simulink model "FBBSC_7dof"  (R2024a)
settings: Solver=ode4  StartTime=0.0  StopTime=20  FixedStep=0.01  RelTol=1e-3
model workspace (MAT data in the model file):
  e2 = Simulink.Signal
  e2.DataType = 'auto'
  e2.Dimensions = [4 1]
  e2.DimensionsMode = 'Fixed'
  e2.Complexity = 'auto'
  e2.SampleTime = -1
  e2.SamplingMode = 'auto'
libraries: aerolibconvert2 x20
settings Model: Creator=hp  LastModifiedBy=somesh
settings SolverCC: ZeroCrossAlgorithm=Adaptive
settings DataIOCC: ReturnWorkspaceOutputs=off
settings DebuggingCC: IgnoredZcDiagnostic=none  UnderSpecifiedDimensionMsg=warning
settings RTWCC: GPUComputeCapability=3.5

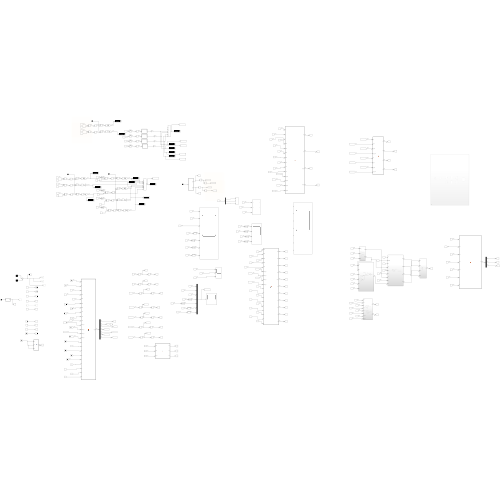
[thumbnail: Simulink's stored preview of the top-level diagram]
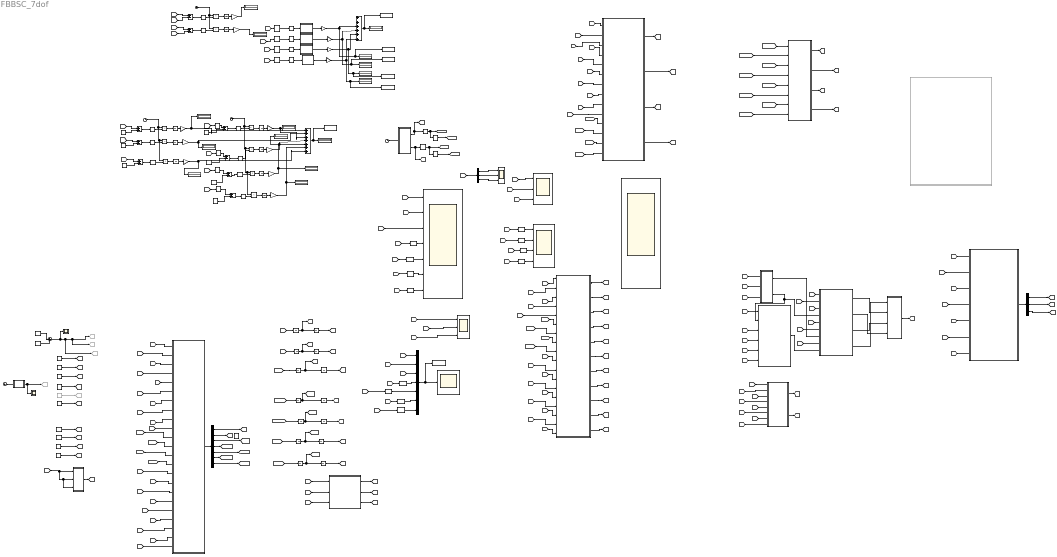
== system FBBSC_7dof ==
  Abs{,1..12} (13 alike) : Abs  SaturateOnIntegerOverflow=off
  Angle Conversion{,1..19} (20 alike) : aerolibconvert2/Angle Conversion  IU=rad  OU=deg
  Clock{,1,5,7..8} (5 alike) : Clock
  Constant : Constant  Value=6.1
  Constant1 : Constant  Value=15.6
  Constant11 : Constant  Value=0.5
  Constant12 : Constant  Value=0.6
  Constant{6..8,13,48..49} (6 alike) : Constant  Value=0
  Constant15 : Constant  Value=0.38
  Constant16 : Constant  Value=6.5
  Constant17 : Constant  Value=0.62
  Constant2 : Constant  Value=2
  Constant3 : Constant
  Constant4 : Constant  Commented=on  Value=0.5
  Constant5 : Constant  Value=0.5
  Constant9 : Constant  Value=0.7
  Demux : Demux  Outputs=7
  Demux1 : Demux  Outputs=3
  Demux3 : Demux  Outputs=3
  Derivative{,1..3} (4 alike) : Derivative
  Display{1..4,25,28..29,39,53..59} (15 alike) : Display
  Gain{,1..12} (13 alike) : Gain
  Goto18 : Goto  Commented=on  GotoTag=Fx
  Goto19 : Goto  Commented=on  GotoTag=Fy
  Goto24 : Goto  Commented=on  GotoTag=l1
  Goto52 : Goto  Commented=on  GotoTag=Fz
  Goto61 : Goto  Commented=on  GotoTag=m2
  Integrator{,1..7,12..20,22} (18 alike) : Integrator
  Integrator{8..11} (4 alike) : Integrator  WrapState=on  WrappedStateUpperValue=pi/2  WrappedStateLowerValue=-pi/2
  Integrator21 : Integrator  InitialCondition=0.5
  MATLAB Function : MATLAB Function  TreatAsAtomicUnit=on
  MATLAB Function1 : MATLAB Function  TreatAsAtomicUnit=on
  MATLAB Function13 : MATLAB Function  TreatAsAtomicUnit=on
  MATLAB Function14 : MATLAB Function  TreatAsAtomicUnit=on
  MATLAB Function16 : MATLAB Function  TreatAsAtomicUnit=on
  MATLAB Function17 : MATLAB Function  TreatAsAtomicUnit=on
  MATLAB Function2 : MATLAB Function  TreatAsAtomicUnit=on
  MATLAB Function20 : MATLAB Function  TreatAsAtomicUnit=on
  MATLAB Function3 : MATLAB Function  TreatAsAtomicUnit=on
  MATLAB Function4 : MATLAB Function  TreatAsAtomicUnit=on
  MATLAB Function5 : MATLAB Function  TreatAsAtomicUnit=on
  MATLAB Function6 : MATLAB Function  TreatAsAtomicUnit=on
  MATLAB Function7 : MATLAB Function  TreatAsAtomicUnit=on
  Mux12 : Mux  Inputs=7
  Product{,1..8} (9 alike) : Product
  Pulse Generator : DiscretePulseGenerator  PulseType=Time based  Amplitude=20  Period=100  PhaseDelay=1
  Pulse Generator1 : DiscretePulseGenerator  PulseType=Time based  Amplitude=-20  Period=100  PhaseDelay=2
  Scope : Scope  NumInputPorts=7
  Scope1 : Scope
  Scope13 : Scope
  Scope2 : Scope
  Scope3 : Scope  NumInputPorts=3
  Scope4 : Scope  NumInputPorts=3
  Scope5 : Scope  NumInputPorts=7
  Scope6 : Scope  NumInputPorts=4
  Scope9 : Scope  NumInputPorts=3
  Subsystem : Subsystem
  Subsystem1 : Subsystem
  Subsystem2 : Subsystem
  Subsystem3 : Subsystem
  Subsystem4 : Subsystem
  Subsystem5 : Subsystem  Commented=on
  Subtract{1..5,16..17,19..20} (9 alike) : Sum  Inputs=+-
  Sum : Sum  Inputs=|+++++++
  Sum2 : Sum  Inputs=|++
  Sum4 : Sum  Inputs=|++++++
  To Workspace : ToWorkspace  VariableName=theta_m  SampleTime=-1
  To Workspace1 : ToWorkspace  VariableName=ITAE  SampleTime=-1
  To Workspace2 : ToWorkspace  VariableName=theta_m1  SampleTime=-1
  To Workspace20 : ToWorkspace  VariableName=values  SaveFormat=Timeseries  SampleTime=-1
  To Workspace3 : ToWorkspace  VariableName=theta_m2  SampleTime=-1
  To Workspace4 : ToWorkspace  VariableName=theta_m3  SampleTime=-1
  To Workspace5 : ToWorkspace  VariableName=theta_m4  SampleTime=-1
  wires:
  [x_ddot] -> Integrator/1
  Integrator/1 -> Integrator6/1, [x_dot]
  [y_ddot] -> Integrator1/1
  Integrator1/1 -> Integrator7/1, [y_dot]
  [theta1_ddot] -> Integrator2/1
  Integrator2/1 -> Integrator8/1, [theta1_dot]
  [theta2_ddot] -> Integrator3/1
  Integrator3/1 -> Integrator9/1, [theta2_dot]
  [theta3_ddot] -> Integrator4/1
  Integrator4/1 -> Integrator10/1, [theta3_dot]
  [theta4_ddot] -> Integrator5/1
  Integrator5/1 -> Integrator11/1, [theta4_dot]
  Integrator6/1 -> [x]
  Integrator7/1 -> [y]
  Integrator8/1 -> [theta1]
  Integrator9/1 -> [theta2]
  Integrator10/1 -> [theta3]
  Integrator11/1 -> [theta4]
  [theta1] -> MATLAB Function/4(theta1)
  [theta2] -> MATLAB Function/5(theta2)
  [theta3] -> MATLAB Function/6(theta3)
  [theta4] -> MATLAB Function/7(theta4)
  [theta1_dot] -> MATLAB Function/11(theta1_dot)
  [theta2_dot] -> MATLAB Function/12(theta2_dot)
  [theta3_dot] -> MATLAB Function/13(theta3_dot)
  [theta4_dot] -> MATLAB Function/14(theta4_dot)
  Pulse Generator1/1 -> Sum2/2
  Pulse Generator/1 -> Sum2/1
  Sum2/1 -> Scope1/1, Goto52/1, Goto19/1, Goto18/1
  [m1] -> MATLAB Function/15(m1)
  [m2] -> MATLAB Function/16(m2)
  [M1] -> MATLAB Function/17(M1)
  [M2] -> MATLAB Function/18(M2)
  [l1] -> MATLAB Function/19(l1)
  [l2] -> MATLAB Function/20(l2)
  Constant/1 -> [M1]
  Constant1/1 -> [M2]
  Constant2/1 -> [m1]
  Constant3/1 -> [m2]
  Constant4/1 -> Goto24/1
  Constant5/1 -> [l2]
  Subtract16/1 -> Abs/1
  Integrator13/1 -> Gain3/1
  Constant7/1 -> Subtract20/2
  Gain2/1 -> Sum/3, Display39/1
  Integrator15/1 -> Gain5/1
  Gain1/1 -> Display25/1, Sum/2
  Product1/1 -> Integrator17/1
  Abs/1 -> Product/2
  [y] -> Subtract17/1
  Product2/1 -> Integrator14/1
  Subtract20/1 -> Abs4/1
  Abs2/1 -> Product2/2
  Abs3/1 -> Product3/2
  Gain5/1 -> Sum/6, Display29/1
  Abs5/1 -> Product5/2
  Integrator17/1 -> Gain1/1
  Clock8/1 -> Product5/1, Product2/1, Product4/1, Product3/1
  Gain3/1 -> Display1/1, Sum/4
  Subtract1/1 -> Abs2/1
  Constant48/1 -> Subtract1/2
  Integrator16/1 -> Gain/1
  Gain/1 -> Sum/1, Display3/1
  Product4/1 -> Integrator13/1
  Integrator14/1 -> Gain4/1
  Constant6/1 -> Subtract19/2
  Integrator12/1 -> Gain2/1
  Constant12/1 -> Subtract17/2
  Product5/1 -> Integrator15/1
  Subtract2/1 -> Abs5/1
  Abs4/1 -> Product4/2
  Product/1 -> Integrator16/1
  Gain4/1 -> Display28/1, Sum/5
  [x] -> Subtract16/1
  Constant49/1 -> Subtract2/2
  Subtract17/1 -> Abs1/1
  Constant11/1 -> Subtract16/2
  Sum/1 -> Display4/1, To Workspace1/1
  Product3/1 -> Integrator12/1
  Abs1/1 -> Product1/2
  [theta2] -> Angle Conversion9/1
  Gain11/1 -> Sum4/6, To Workspace5/1, Display56/1
  Subtract4/1 -> Abs7/1
  Gain10/1 -> To Workspace4/1, Display58/1, Sum4/5
  Subtract3/1 -> Abs6/1
  Abs11/1 -> MATLAB Function2/1(u)
  MATLAB Function20/1(y) -> Gain11/1
  [x_d] -> Subtract3/2
  [y_d] -> Subtract4/2
  [x] -> Subtract3/1
  MATLAB Function2/1(y) -> Gain8/1
  [theta4] -> Angle Conversion11/1
  Clock5/1 -> Product7/1, Product6/1
  MATLAB Function16/1(y) -> Gain10/1
  [theta3] -> Angle Conversion10/1
  Abs6/1 -> Product6/2
  [y] -> Subtract4/1
  Abs9/1 -> MATLAB Function16/1(u)
  Integrator18/1 -> Gain6/1
  Sum4/1 -> To Workspace/1, Display59/1
  Abs10/1 -> MATLAB Function20/1(u)
  MATLAB Function13/1(y) -> Gain9/1
  Product7/1 -> Integrator19/1
  Abs8/1 -> MATLAB Function13/1(u)
  [theta1] -> Angle Conversion8/1
  Gain7/1 -> Display54/1
  Product6/1 -> Integrator18/1
  Gain6/1 -> Display57/1
  Abs7/1 -> Product7/2
  Gain9/1 -> Sum4/4, To Workspace3/1, Display55/1
  Integrator19/1 -> Gain7/1
  Subtract19/1 -> Abs3/1
  [theta1] -> Angle Conversion4/1
  Angle Conversion4/1 -> Subtract19/1
  [theta2] -> Angle Conversion5/1
  Angle Conversion5/1 -> Subtract20/1
  [theta3] -> Angle Conversion6/1
  Angle Conversion6/1 -> Subtract1/1
  [theta4] -> Angle Conversion7/1
  Angle Conversion7/1 -> Subtract2/1
  Angle Conversion8/1 -> Abs11/1
  Angle Conversion9/1 -> Abs8/1
  Angle Conversion10/1 -> Abs9/1
  Angle Conversion11/1 -> Abs10/1
  [theta3] -> Angle Conversion16/1
  [theta1] -> Angle Conversion14/1
  Mux12/1 -> Scope2/1, To Workspace20/1
  [theta2] -> Angle Conversion15/1
  [theta4] -> Angle Conversion17/1
  [x] -> Scope/1
  [y] -> Scope/2
  [theta4] -> Angle Conversion3/1
  [theta3] -> Angle Conversion2/1
  [theta1] -> Angle Conversion/1
  [theta2] -> Angle Conversion1/1
  [x] -> MATLAB Function3/1(x)
  [y] -> MATLAB Function3/2(y)
  [theta1] -> MATLAB Function3/4(theta1)
  [theta2] -> MATLAB Function3/5(theta2)
  [theta3] -> MATLAB Function3/6(theta3)
  [theta4] -> MATLAB Function3/7(theta4)
  [x_dot] -> MATLAB Function3/8(x_dot)
  [y_dot] -> MATLAB Function3/9(y_dot)
  [theta1_dot] -> MATLAB Function3/11(theta1_dot)
  [theta2_dot] -> MATLAB Function3/12(theta2_dot)
  [theta3_dot] -> MATLAB Function3/13(theta3_dot)
  [theta4_dot] -> MATLAB Function3/14(theta4_dot)
  MATLAB Function3/1(qx) -> [qx]
  MATLAB Function3/2(qs) -> [qs]
  MATLAB Function3/3(qx_dot) -> [qx_dot]
  MATLAB Function3/4(qs_dot) -> [qs_dot]
  [qx_dot] -> MATLAB Function5/7(qx_dot)
  MATLAB Function5/3(e3) -> [e3]
  [qs_dot] -> MATLAB Function5/3(qs_dot)
  [qs_d] -> MATLAB Function5/2(qs_d)
  [qx] -> MATLAB Function5/5(qx)
  MATLAB Function5/4(e4) -> [e4]
  MATLAB Function5/2(e2) -> [e2]
  [qx_d] -> MATLAB Function5/6(qx_d)
  MATLAB Function5/1(e1) -> [e1]
  [qs_d_Dot] -> MATLAB Function5/4(qs_d_dot)
  [qs] -> MATLAB Function5/1(qs)
  [qx_d_Dot] -> MATLAB Function5/8(qx_d_dot)
  [Fx] -> MATLAB Function/1(Fx)
  [Fy] -> MATLAB Function/2(Fy)
  MATLAB Function/1(q_ddot) -> Demux/1
  [x_dot] -> MATLAB Function/8(x_dot)
  [y_dot] -> MATLAB Function/9(y_dot)
  [e3] -> Subsystem1/5(e3)
  MATLAB Function14/4(mss) -> [mss]
  MATLAB Function14/5(mss_I) -> [mss_I]
  MATLAB Function14/3(msx) -> [msx]
  MATLAB Function14/6(cxx) -> [cxx]
  [theta1_dot] -> MATLAB Function14/6(theta1_dot)
  [theta2_dot] -> MATLAB Function14/7(theta2_dot)
  [m1] -> MATLAB Function14/10(m1)
  [m2] -> MATLAB Function14/11(m2)
  [theta4] -> MATLAB Function14/4(theta4)
  [theta1] -> MATLAB Function14/1(theta1)
  [l2] -> MATLAB Function14/15(l2)
  MATLAB Function14/11(G2) -> [G2]
  MATLAB Function14/2(mxs) -> [mxs]
  [K] -> Subsystem/8(K)
  [M2] -> MATLAB Function14/13(M2)
  MATLAB Function14/8(csx) -> [csx]
  [K] -> Subsystem1/4(K)
  Subsystem/2(T4) -> Subsystem2/4(T4)
  MATLAB Function14/10(G1) -> [G1]
  [theta4_dot] -> MATLAB Function14/9(theta4_dot)
  [e2] -> Subsystem/6(e2)
  MATLAB Function14/7(cxs) -> [cxs]
  [qs_dot] -> Subsystem3/8(qs_dot)
  Subsystem4/1(ff) -> Subsystem/7(ff)
  Subsystem3/1(hx) -> [hx]
  Subsystem/3(T3) -> Subsystem2/3(T3)
  [theta3] -> MATLAB Function14/3(theta3)
  [css] -> Subsystem3/5(css)
  Subsystem/1(T2) -> Subsystem2/2(T2)
  [e4] -> Subsystem1/3(e4)
  [lambda] -> Subsystem/2(lambda)
  MATLAB Function14/9(css) -> [css]
  [G2] -> Subsystem3/6(G2)
  Subsystem/4(T1) -> Subsystem2/1(T1)
  [G1] -> Subsystem3/3(G1)
  Subsystem3/2(hs) -> [hs]
  MATLAB Function14/1(mxx) -> [mxx]
  [csx] -> Subsystem3/4(csx)
  [c2] -> Subsystem/3(c2)
  [l1] -> MATLAB Function14/14(l1)
  [qx_dot] -> Subsystem3/7(qx_dot)
  [e1] -> Subsystem1/6(e1)
  Subsystem2/1(U) -> [U]
  [cxx] -> Subsystem3/1(cxx)
  [hs] -> Subsystem4/2(hs)
  Subsystem1/1(z1) -> Subsystem/9(z1)
  [msx] -> Subsystem4/3(msx)
  [e4] -> Subsystem/5(e4)
  [mss_I] -> Subsystem4/1(mss_I)
  [M1] -> MATLAB Function14/12(M1)
  [e2] -> Subsystem1/1(e2)
  [mxx] -> MATLAB Function17/2(mxx)
  [U] -> MATLAB Function17/1(U)
  [msx] -> MATLAB Function17/5(msx)
  [c1] -> Subsystem/1(c1)
  MATLAB Function17/1(tau) -> Demux1/1
  [hs] -> MATLAB Function17/7(hs)
  [mss] -> MATLAB Function17/4(mss)
  Subsystem4/2(gf) -> Subsystem/4(gf), Subsystem1/2(gf)
  [theta2] -> MATLAB Function14/2(theta2)
  [theta3_dot] -> MATLAB Function14/8(theta3_dot)
  [mxs] -> MATLAB Function17/3(mxs)
  [cxs] -> Subsystem3/2(cxs)
  [hx] -> MATLAB Function17/6(hx)
  Gain8/1 -> To Workspace2/1, Display53/1, Sum4/3
  [Fx] -> Scope3/1
  [Fy] -> Scope3/2
  MATLAB Function1/1(K) -> [K]
  MATLAB Function4/1(m2) -> Goto61/1, Scope13/1
  Clock1/1 -> MATLAB Function4/1(t)
  [k] -> MATLAB Function1/3(k3), MATLAB Function1/2(k2), MATLAB Function1/1(k1)
  [x_dot] -> MATLAB Function7/1(x_dot)
  [y_dot] -> MATLAB Function7/2(y_dot)
  MATLAB Function7/1(Frx) -> [Frx]
  MATLAB Function7/2(Fry) -> [Fry]
  [Frx] -> MATLAB Function/21(Frx)
  [Fry] -> MATLAB Function/22(Fry)
  [Frx] -> MATLAB Function14/16(Frx)
  [Fry] -> MATLAB Function14/17(Fry)
  Constant15/1 -> [c1]
  Constant16/1 -> [c2]
  Constant17/1 -> [k]
  Constant13/1 -> [lambda]
  [Frz] -> MATLAB Function14/18(Frz)
  [Fz] -> MATLAB Function/3(Fz)
  [l1_dot] -> MATLAB Function7/3(l1_dot)
  MATLAB Function7/3(Frz) -> [Frz]
  Demux/7 -> [theta4_ddot]
  Demux/6 -> [theta3_ddot]
  Demux/5 -> [theta2_ddot]
  Demux/4 -> [theta1_ddot]
  Demux/2 -> [y_ddot]
  Demux/1 -> [x_ddot]
  [l1_dot] -> MATLAB Function/10(l1_dot)
  [Frz] -> MATLAB Function/23(Frz)
  [l1_ddot] -> Integrator20/1
  Integrator20/1 -> [l1_dot], Integrator21/1
  Integrator21/1 -> [l1]
  [Fz] -> Scope3/3
  [x] -> Mux12/1
  [y] -> Mux12/2
  [l1] -> Mux12/3
  Angle Conversion14/1 -> Mux12/4
  Angle Conversion15/1 -> Mux12/5
  Angle Conversion16/1 -> Mux12/6
  Angle Conversion17/1 -> Mux12/7
  [l1_dot] -> MATLAB Function14/5(l1_dot)
  [l1] -> Scope/3
  Angle Conversion/1 -> Scope/4
  Angle Conversion1/1 -> Scope/5
  Angle Conversion2/1 -> Scope/6
  Angle Conversion3/1 -> Scope/7
  [l1] -> MATLAB Function3/3(l)
  [l1_dot] -> MATLAB Function3/10(l_dot)
  Demux1/1 -> [Fx]
  Demux1/2 -> [Fy]
  Demux1/3 -> [Fz]
  Demux/3 -> [l1_ddot]
  Abs12/1 -> Product8/2
  Subtract5/1 -> Abs12/1
  Constant9/1 -> Subtract5/2
  Clock7/1 -> Product8/1, Product1/1, Product/1
  Integrator22/1 -> Gain12/1
  [l1] -> Subtract5/1
  Product8/1 -> Integrator22/1
  Gain12/1 -> Sum/7, Display2/1
  [theta1] -> Angle Conversion12/1
  [theta2] -> Angle Conversion13/1
  [theta3] -> Angle Conversion18/1
  [theta4] -> Angle Conversion19/1
  [x] -> Scope4/1
  [y] -> Scope4/2
  [l1] -> Scope4/3
  Angle Conversion12/1 -> Scope6/1
  Angle Conversion13/1 -> Scope6/2
  Angle Conversion18/1 -> Scope6/3
  Angle Conversion19/1 -> Scope6/4
  Demux3/3 -> Scope9/3
  [qx_d] -> Demux3/1
  Derivative1/1 -> [qs_d_DDot]
  Derivative2/1 -> Derivative3/1, [qx_d_Dot]
  MATLAB Function6/1(qs_d) -> Derivative/1, [qs_d]
  Demux3/1 -> Scope9/1
  Demux3/2 -> Scope9/2
  Clock/1 -> MATLAB Function6/1(t)
  Derivative/1 -> Derivative1/1, [qs_d_Dot]
  Derivative3/1 -> [qx_d_DDot]
  MATLAB Function6/2(qx_d) -> [qx_d], Derivative2/1

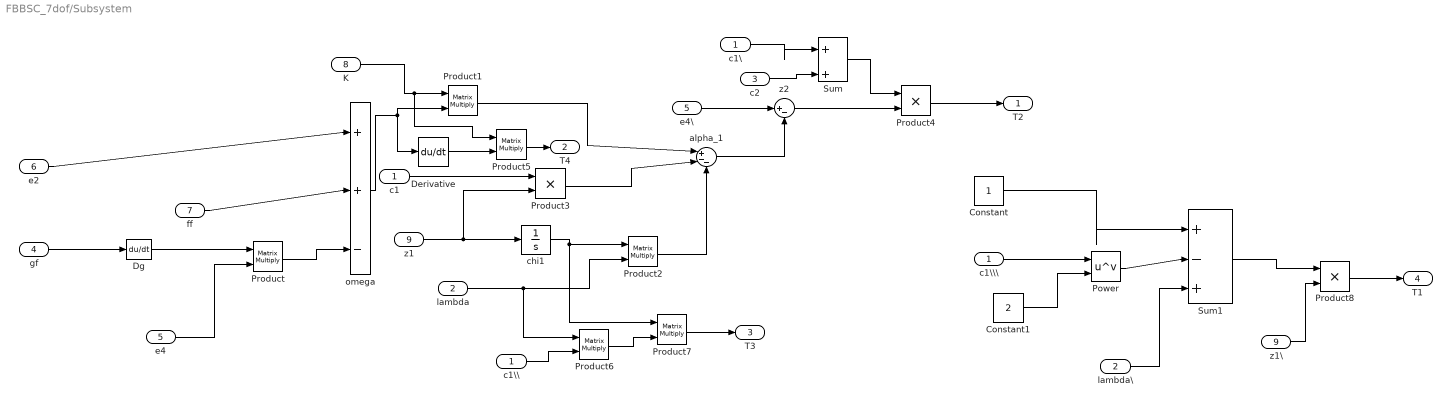
== system FBBSC_7dof/Subsystem ==
  c1 : Inport
  lambda : Inport  Port=2
  c2 : Inport  Port=3
  gf : Inport  Port=4  PortDimensions=[4 3]
  e4 : Inport  Port=5  PortDimensions=[3 1]
  e2 : Inport  Port=6  PortDimensions=[4 1]
  ff : Inport  Port=7  PortDimensions=[4 1]
  K : Inport  Port=8  PortDimensions=[3 4]
  z1 : Inport  Port=9  PortDimensions=[3 1]
  Constant : Constant
  Constant1 : Constant  Value=2
  Derivative : Derivative
  Dg : Derivative
  Power : Math  Operator=pow
  Product{,1..2,5..7} (6 alike) : Product  Multiplication=Matrix(*)
  Product3 : Product
  Product4 : Product
  Product8 : Product
  Sum : Sum  Inputs=|++
  Sum1 : Sum  Inputs=|+-+
  alpha_1 : Sum  Inputs=|+--
  c1\ : InportShadow
  c1\\ : InportShadow
  c1\\\ : InportShadow
  chi1 : Integrator
  e4\ : InportShadow  Port=5  PortDimensions=[3 1]
  lambda\ : InportShadow  Port=2
  omega : Sum  Inputs=|++-
  z1\ : InportShadow  Port=9  PortDimensions=[3 1]
  z2 : Sum  Inputs=|+-
  T2 : Outport  PortDimensions=[3 1]
  T4 : Outport  Port=2  PortDimensions=[3 1]
  T3 : Outport  Port=3  PortDimensions=[3 1]
  T1 : Outport  Port=4  PortDimensions=[3 1]
  wires:
  Dg/1 -> Product/1
  Product/1 -> omega/3
  omega/1 -> Product1/2, Derivative/1
  chi1/1 -> Product7/1, Product2/1
  lambda/1 -> Product6/1, Product2/2
  c1/1 -> Product3/1
  Product1/1 -> alpha_1/1
  Product3/1 -> alpha_1/2
  Product2/1 -> alpha_1/3
  alpha_1/1 -> z2/2
  c1\/1 -> Sum/1
  c2/1 -> Sum/2
  Sum/1 -> Product4/1
  z2/1 -> Product4/2
  Product4/1 -> T2/1
  Derivative/1 -> Product5/2
  Product5/1 -> T4/1
  c1\\/1 -> Product6/2
  Product6/1 -> Product7/2
  Product7/1 -> T3/1
  c1\\\/1 -> Power/1
  Constant1/1 -> Power/2
  Constant/1 -> Sum1/1
  Power/1 -> Sum1/2
  lambda\/1 -> Sum1/3
  Sum1/1 -> Product8/1
  Product8/1 -> T1/1
  gf/1 -> Dg/1
  e4/1 -> Product/2
  e2/1 -> omega/1
  ff/1 -> omega/2
  K/1 -> Product5/1, Product1/1
  z1/1 -> chi1/1, Product3/2
  e4\/1 -> z2/1
  z1\/1 -> Product8/2

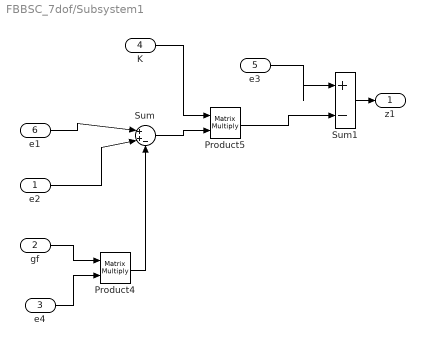
== system FBBSC_7dof/Subsystem1 ==
  e2 : Inport  PortDimensions=[4 1]
  gf : Inport  Port=2  PortDimensions=[4 3]
  e4 : Inport  Port=3  PortDimensions=[3 1]
  K : Inport  Port=4  PortDimensions=[3 4]
  e3 : Inport  Port=5  PortDimensions=[3 1]
  e1 : Inport  Port=6  PortDimensions=[4 1]
  Product4 : Product  Multiplication=Matrix(*)
  Product5 : Product  Multiplication=Matrix(*)
  Sum : Sum  Inputs=|++-
  Sum1 : Sum  Inputs=|+-
  z1 : Outport  PortDimensions=[3 1]
  wires:
  K/1 -> Product5/1
  gf/1 -> Product4/1
  e3/1 -> Sum1/1
  Product5/1 -> Sum1/2
  Sum/1 -> Product5/2
  e2/1 -> Sum/2
  e1/1 -> Sum/1
  e4/1 -> Product4/2
  Product4/1 -> Sum/3
  Sum1/1 -> z1/1

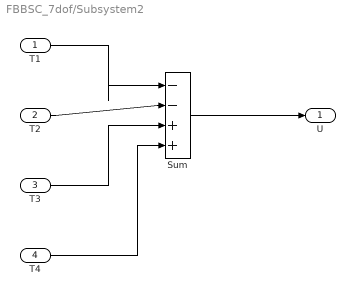
== system FBBSC_7dof/Subsystem2 ==
  T1 : Inport  PortDimensions=[3 1]
  T2 : Inport  Port=2  PortDimensions=[3 1]
  T3 : Inport  Port=3  PortDimensions=[3 1]
  T4 : Inport  Port=4  PortDimensions=[3 1]
  Sum : Sum  Inputs=|--++
  U : Outport  PortDimensions=[3 1]
  wires:
  T1/1 -> Sum/1
  T2/1 -> Sum/2
  T3/1 -> Sum/3
  T4/1 -> Sum/4
  Sum/1 -> U/1

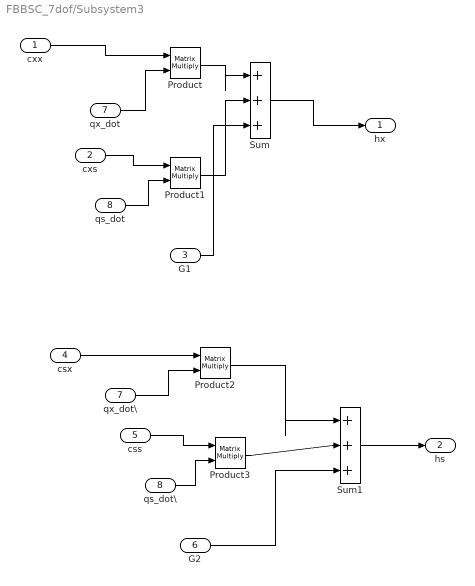
== system FBBSC_7dof/Subsystem3 ==
  cxx : Inport  PortDimensions=[3 3]
  cxs : Inport  Port=2  PortDimensions=[3 4]
  G1 : Inport  Port=3  PortDimensions=[3 1]
  csx : Inport  Port=4  PortDimensions=[4 3]
  css : Inport  Port=5  PortDimensions=[4 4]
  G2 : Inport  Port=6  PortDimensions=[4 1]
  qx_dot : Inport  Port=7  PortDimensions=[3 1]
  qs_dot : Inport  Port=8  PortDimensions=[4 1]
  Product{,1..3} (4 alike) : Product  Multiplication=Matrix(*)
  Sum : Sum  Inputs=|+++
  Sum1 : Sum  Inputs=|+++
  qs_dot\ : InportShadow  Port=8  PortDimensions=[4 1]
  qx_dot\ : InportShadow  Port=7  PortDimensions=[3 1]
  hx : Outport  PortDimensions=[3 1]
  hs : Outport  Port=2  PortDimensions=[4 1]
  wires:
  cxx/1 -> Product/1
  qx_dot/1 -> Product/2
  cxs/1 -> Product1/1
  qs_dot/1 -> Product1/2
  Product/1 -> Sum/1
  Product1/1 -> Sum/2
  G1/1 -> Sum/3
  Sum/1 -> hx/1
  Sum1/1 -> hs/1
  csx/1 -> Product2/1
  qx_dot\/1 -> Product2/2
  Product2/1 -> Sum1/1
  css/1 -> Product3/1
  qs_dot\/1 -> Product3/2
  Product3/1 -> Sum1/2
  G2/1 -> Sum1/3

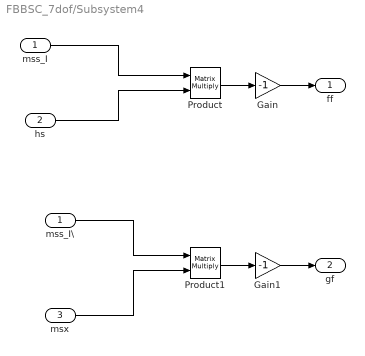
== system FBBSC_7dof/Subsystem4 ==
  mss_I : Inport  PortDimensions=[4 4]
  hs : Inport  Port=2  PortDimensions=[4 1]
  msx : Inport  Port=3  PortDimensions=[4 3]
  Gain : Gain  Gain=-1
  Gain1 : Gain  Gain=-1
  Product : Product  Multiplication=Matrix(*)
  Product1 : Product  Multiplication=Matrix(*)
  mss_I\ : InportShadow  PortDimensions=[4 4]
  ff : Outport  PortDimensions=[4 1]
  gf : Outport  Port=2  PortDimensions=[4 3]
  wires:
  hs/1 -> Product/2
  msx/1 -> Product1/2
  Product/1 -> Gain/1
  mss_I/1 -> Product/1
  mss_I\/1 -> Product1/1
  Product1/1 -> Gain1/1
  Gain/1 -> ff/1
  Gain1/1 -> gf/1

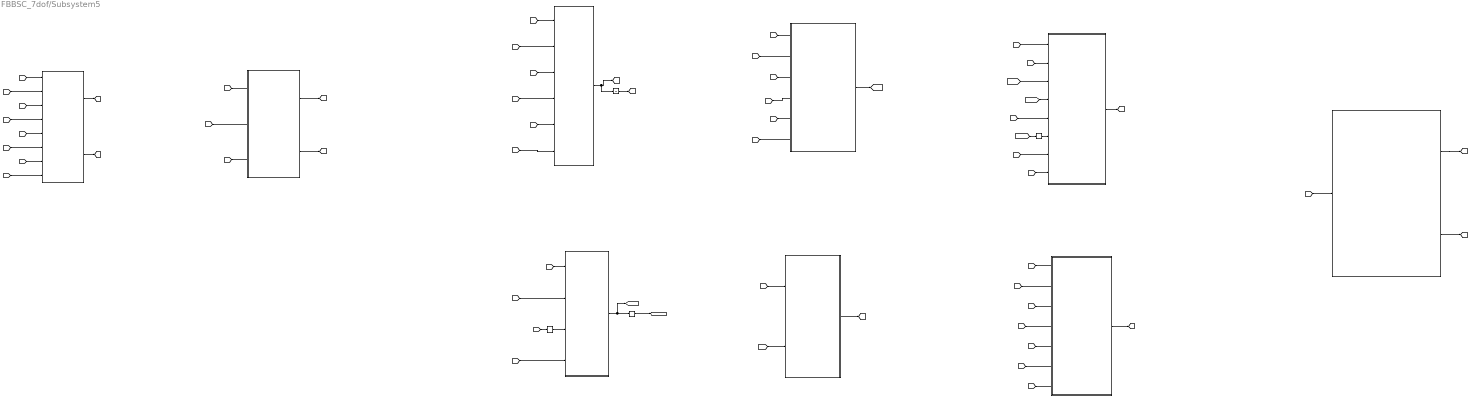
== system FBBSC_7dof/Subsystem5 ==
  Derivative4 : Derivative
  Integrator20 : Integrator
  MATLAB Function1 : MATLAB Function  TreatAsAtomicUnit=on
  MATLAB Function10 : MATLAB Function  TreatAsAtomicUnit=on
  MATLAB Function11 : MATLAB Function  TreatAsAtomicUnit=on
  MATLAB Function12 : MATLAB Function  TreatAsAtomicUnit=on
  MATLAB Function15 : MATLAB Function  TreatAsAtomicUnit=on
  MATLAB Function4 : MATLAB Function  TreatAsAtomicUnit=on
  MATLAB Function7 : MATLAB Function  TreatAsAtomicUnit=on
  MATLAB Function8 : MATLAB Function  TreatAsAtomicUnit=on
  MATLAB Function9 : MATLAB Function  TreatAsAtomicUnit=on
  Memory : Memory
  Memory3 : Memory
  wires:
  [c1] -> MATLAB Function11/1(c1)
  [z2] -> MATLAB Function11/4(z2)
  [lambda] -> MATLAB Function11/7(lambda)
  [msx] -> MATLAB Function12/5(msx)
  [chi1] -> MATLAB Function11/5(chi1)
  [Va] -> MATLAB Function15/1(tau)
  MATLAB Function8/1(Omega) -> Derivative4/1, [Omega]
  [c2] -> MATLAB Function11/2(c2)
  Memory/1 -> MATLAB Function11/6(omega_dot)
  [e2] -> MATLAB Function7/2(e2)
  [z1] -> MATLAB Function11/3(z1)
  [e4] -> MATLAB Function10/1(e4)
  MATLAB Function10/1(z2) -> [z2]
  [Dg] -> Memory3/1
  [Omega_dot] -> Memory/1
  [gf] -> MATLAB Function7/5(gf)
  [Omega] -> MATLAB Function9/6(Omega)
  Derivative4/1 -> [Omega_dot]
  [k] -> MATLAB Function7/6(k)
  MATLAB Function7/1(z1) -> Integrator20/1, [z1]
  [mxx] -> MATLAB Function12/2(mxx)
  [e4] -> MATLAB Function7/4(e4)
  [z1] -> MATLAB Function9/2(z1)
  [alpha_1] -> MATLAB Function10/2(alpha_1)
  MATLAB Function9/1(alpha_1) -> [alpha_1]
  MATLAB Function12/1(tau) -> [Va]
  MATLAB Function15/2(Fy) -> [Fy]
  [mxs] -> MATLAB Function12/3(mxs)
  [e1] -> MATLAB Function7/1(e1)
  Memory3/1 -> MATLAB Function8/3(Dg)
  MATLAB Function15/1(Fx) -> [Fx]
  [mss] -> MATLAB Function12/4(mss)
  MATLAB Function11/1(U) -> [U]
  Integrator20/1 -> [chi1]
  [ff] -> MATLAB Function8/2(ff)
  [k] -> MATLAB Function11/8(k)
  [e4] -> MATLAB Function8/4(e4)
  [e2] -> MATLAB Function8/1(e2)
  [hx] -> MATLAB Function12/6(hx)
  [e3] -> MATLAB Function7/3(e3)
  [chi1] -> MATLAB Function9/4(chi1)
  [k] -> MATLAB Function9/5(k)
  [lambda] -> MATLAB Function9/3(lambda)
  [hs] -> MATLAB Function12/7(hs)
  [U] -> MATLAB Function12/1(U)
  [c1] -> MATLAB Function9/1(c1)
  [G1] -> MATLAB Function1/3(G1)
  [qx_dot] -> MATLAB Function1/7(qx_dot)
  [msx] -> MATLAB Function4/2(msx)
  [csx] -> MATLAB Function1/4(csx)
  MATLAB Function4/1(ff) -> [ff]
  MATLAB Function4/2(gf) -> [gf]
  [qs_dot] -> MATLAB Function1/8(qs_dot)
  [mss] -> MATLAB Function4/1(mss)
  [css] -> MATLAB Function1/5(css)
  [cxs] -> MATLAB Function1/2(cxs)
  [hs] -> MATLAB Function4/3(hs)
  [G2] -> MATLAB Function1/6(G2)
  MATLAB Function1/2(hs) -> [hs]
  MATLAB Function1/1(hx) -> [hx]
  [cxx] -> MATLAB Function1/1(cxx)

== matlab function FBBSC_7dof/MATLAB Function13 ==
  settings: updateMethod=DISCRETE
  data: u input; y output
function y = fcn(u)
    persistent maxVal;
    
    % Check if maxVal is empty and initialize it if necessary
    if isempty(maxVal)
        maxVal = 0; % Initialize with negative infinity or another suitable value
    end
    
    % Update maxVal if the current input is greater
    if u > maxVal
        maxVal = u;
    end
    
    y = maxVal;
end

== matlab function FBBSC_7dof/MATLAB Function3 ==
  data: x input; qx output size=[3 1]; y input; l input; theta1 input; theta2 input; theta3 input; theta4 input; x_dot input; y_dot input; l_dot input; theta1_dot input; theta2_dot input; theta3_dot input; theta4_dot input; qs output size=[4 1]; qx_dot output size=[3 1]; qs_dot output size=[4 1]
function [qx, qs, qx_dot, qs_dot] = fcn(x, y, l, theta1, theta2, theta3, theta4,...
    x_dot, y_dot, l_dot, theta1_dot, theta2_dot, theta3_dot, theta4_dot)

qx = [x;y;l];
qs = [theta1;theta2;theta3;theta4];
qx_dot = [x_dot;y_dot; l_dot];
qs_dot = [theta1_dot;theta2_dot;theta3_dot;theta4_dot];

end

== matlab function FBBSC_7dof/Subsystem5/MATLAB Function4 ==
  data: mss input; ff output; msx input; hs input; gf output
function [ff, gf] = fcn(mss, msx, hs)

ff = -inv(mss)*hs;
gf = -inv(mss)*msx;

end

== matlab function FBBSC_7dof/MATLAB Function5 ==
  data: qs input size=[4 1]; e1 output size=[4 1]; qs_d input size=[4 1]; qs_dot input size=[4 1]; qs_d_dot input size=[4 1]; qx input size=[3 1]; qx_d input size=[3 1]; qx_dot input size=[3 1]; qx_d_dot input size=[3 1]; e2 output size=[4 1]; e3 output size=[3 1]; e4 output size=[3 1]
function [e1, e2, e3, e4] = fcn(qs, qs_d, qs_dot, qs_d_dot, qx, qx_d, qx_dot, qx_d_dot)


e1 = qs - qs_d;
e2 = qs_dot - qs_d_dot;
e3 = qx - qx_d;
e4 = qx_dot - qx_d_dot;

end

== matlab function FBBSC_7dof/MATLAB Function6 ==
  data: t input; qs_d output; qx_d output
function [qs_d, qx_d] = fcn(t)

qs_d = zeros(4,1);
qx_d = [0.5;0.6; 0.7];

% x0=0;
% y0=0;
% z0=0;
% x_d=0.5;
% y_d=0.6;
% z_d=0.7;
% kv= 0.4;
% ka = 0.4;
% epsilon = 1.5;
% k1 = (2*ka)/kv;
% k2 = (2*ka)/(kv^2);
% qx_d(1) = x0 + (x_d/2) + (kv/(2*k1))*(sqrt(1+(k1*t - epsilon)^2) - sqrt(1 + (k1*t - epsilon - k2*x_d)^2));
% qx_d(2) = y0 + (y_d/2) + (kv/(2*k1))*(sqrt(1+(k1*t - epsilon)^2) - sqrt(1 + (k1*t - epsilon - k2*y_d)^2));
% qx_d(3) = z0 + (z_d/2) + (kv/(2*k1))*(sqrt(1+(k1*t - epsilon)^2) - sqrt(1 + (k1*t - epsilon - k2*z_d)^2));

end


% if t >= 0 && t <= 20
%     
%   x_d = 0.02*t^2;
%   y_d = 0.03*t^2 ;
% 
%   
% elseif t >= 20 && t <= 60
%     
%   x_d = 8;
%   y_d = 12;
% 
%   
% elseif t >= 60 && t <= 80
%     
%   x_d = 8 + ((t - (60))^2)*0.03;
%   y_d = 12 + ((t-(60))^2)*0.02;
% 
%   
% else
%     x_d = 20;
%     y_d = 20;

== matlab function FBBSC_7dof/Subsystem5/MATLAB Function7 ==
  data: e1 input; z1 output; e2 input; e3 input; e4 input; gf input; k input
function z1  = fcn(e1, e2, e3, e4, gf, k)

K = [k, 0, 0, 0;
    0, k, 0, 0];

z1 = e3 - K*(e1 + e2 - gf*e4);




end

== matlab function FBBSC_7dof/Subsystem5/MATLAB Function8 ==
  data: e2 input; Omega output; ff input; Dg input; e4 input
function Omega = fcn(e2, ff, Dg, e4)

Omega = e2 + ff - Dg*e4;

end

== matlab function FBBSC_7dof/Subsystem5/MATLAB Function9 ==
  data: c1 input; alpha_1 output; z1 input; lambda input; chi1 input; k input; Omega input
function alpha_1 = fcn(c1, z1, lambda, chi1, k, Omega)


K = [k, 0, 0, 0;
    0, k, 0, 0];

alpha_1 = -c1.*z1 - lambda.*chi1 + K*Omega;

end

== matlab function FBBSC_7dof/Subsystem5/MATLAB Function10 ==
  data: e4 input; z2 output; alpha_1 input
function z2 = fcn(e4, alpha_1)

z2 = e4 - alpha_1;

end

== matlab function FBBSC_7dof/Subsystem5/MATLAB Function11 ==
  data: c1 input; c2 input; z1 input size=[2 1]; z2 input size=[2 1]; chi1 input size=[2 1]; omega_dot input size=[4 1]; lambda input; k input; U output size=[2 1]
function U  = fcn(c1, c2, z1, z2, chi1, omega_dot, lambda, k)

K = [k, 0, 0, 0;
    0, k, 0, 0];


U = - (1 - c1^2 + lambda).*z1 - (c1 + c2).*z2 + (lambda*c1).*chi1 + K*omega_dot;

end

== matlab function FBBSC_7dof/Subsystem5/MATLAB Function12 ==
  data: U input size=[2 1]; tau output; mxx input size=[2 2]; mxs input size=[2 4]; mss input size=[4 4]; msx input size=[4 2]; hx input size=[2 1]; hs input size=[4 1]
function tau  = fcn(U, mxx, mxs, mss, msx, hx, hs)

B = [1, 0; 0, 1];

tau = inv(B'*B)*B'*((mxx - mxs*inv(mss)*msx)*U + (hx - mxs*inv(mss)*hs));


end

== matlab function FBBSC_7dof/MATLAB Function14 ==
  data: theta1 input; theta2 input; theta3 input; theta4 input; l1_dot input; theta1_dot input; theta2_dot input; theta3_dot input; theta4_dot input; m1 input; m2 input; M1 input; M2 input; l1 input; l2 input; mxx output; mxs output; msx output; mss output; mss_I output; cxx output; cxs output; csx output; css output; G1 output; G2 output; Frx input; Fry input; Frz input
function [mxx, mxs, msx, mss, mss_I, cxx, cxs, csx, css, G1, G2]   = fcn(theta1, theta2, theta3, theta4,...
    l1_dot, theta1_dot, theta2_dot, theta3_dot, theta4_dot,...
    m1, m2, M1, M2, l1, l2, Frx, Fry, Frz)


g = 9.8;


% Mass matrix M(q)
M = zeros(7, 7);

% Define M matrix elements
M(1,1) = M1 + m1 + m2;
M(1,2) = 0;
M(1,3) = (m1 + m2) * sin(theta1) * cos(theta2);
M(1,4) = (m1 + m2) * l1 * cos(theta1) * cos(theta2);
M(1,5) = -(m1 + m2) * l1 * sin(theta1) * sin(theta2);
M(1,6) = m2 * l2 * cos(theta3) * cos(theta4);
M(1,7) = -m2 * l2 * sin(theta3) * sin(theta4);

M(2,1) = 0;
M(2,2) = M2 + m1 + m2;
M(2,3) = (m1 + m2) * sin(theta2);
M(2,4) = 0;
M(2,5) = (m1 + m2) * l1 * cos(theta2);
M(2,6) = 0;
M(2,7) = m2 * l2 * cos(theta4);

M(3,1) = (m1 + m2) * sin(theta1) * cos(theta2);
M(3,2) = (m1 + m2) * sin(theta2);
M(3,3) = m1 + m2;
M(3,4) = 0;
M(3,5) = 0;
M(3,6) = m2 * l2 * cos(theta2) * cos(theta4) * sin(theta1 - theta3);
M(3,7) = m2 * l2 * (sin(theta2) * cos(theta4) - cos(theta2) * sin(theta4) * cos(theta1 - theta3));

M(4,1) = (m1 + m2) * l1 * cos(theta1) * cos(theta2);
M(4,2) = 0;
M(4,3) = 0;
M(4,4) = (m1 + m2) * l1^2 * cos(theta2)^2;
M(4,5) = 0;
M(4,6) = m2*l1*l2*cos(theta2)*cos(theta4)*cos(theta1-theta3);
M(4,7) = m2*l1*l2*cos(theta2)*sin(theta4)*sin(theta1 - theta3);

M(5,1) = -(m1 + m2) * l1 * sin(theta1) * sin(theta2);
M(5,2) = (m1 + m2) * l1 * cos(theta2);
M(5,3) = 0;
M(5,4) = 0;
M(5,5) = (m1 + m2) * l1^2;
M(5,6) = -m2 * l1 * l2 * sin(theta2) * cos(theta4) * sin(theta1 - theta3);
M(5,7) = m2 * l1 * l2 * (cos(theta2) * cos(theta4) + sin(theta2) * sin(theta4) * cos(theta1 - theta3));

M(6,1) = m2 * l2 * cos(theta3) * cos(theta4);
M(6,2) = 0;
M(6,3) = m2 * l2 * cos(theta2) * cos(theta4) * sin(theta1 - theta3);
M(6,4) = m2*l1*l2*cos(theta2)*cos(theta4)*cos(theta1-theta3);
M(6,5) = -m2 * l1 * l2 * sin(theta2) * cos(theta4) * sin(theta1 - theta3);
M(6,6) = m2 * l2^2 * cos(theta4)^2;
M(6,7) = 0;

M(7,1) = -m2 * l2 * sin(theta3) * sin(theta4);
M(7,2) = m2 * l2 * cos(theta4);
M(7,3) = m2 * l2 * (sin(theta2) * cos(theta4) - cos(theta2) * sin(theta4) * cos(theta1 - theta3));
M(7,4) = m2*l1*l2*cos(theta2)*sin(theta4)*sin(theta1 - theta3);
M(7,5) = m2 * l1 * l2 * (cos(theta2) * cos(theta4) + sin(theta2) * sin(theta4) * cos(theta1 - theta3));
M(7,6) = 0;
M(7,7) = m2 * l2^2;

% spliting

mxx = M(1:3, 1:3);
mxs = M(1:3, 4:7);
msx = M(4:7, 1:3);
mss = M(4:7, 4:7);
mss_I = -inv(mss);

%%%%%%%%%%%%%%%%%%%%%%%%%%%%%%%%%%%%%%%%%%%%%%%%%%%%%%%%%%%%%%%%%%%%%%%%%%%%%%%%%%%%%%%%%%%%%%%%%%%%%%%%%%%%%%%%%%%%%%%%%%%%%%%%%%%%%%%%%%%%%%%%%%%%%%%%%%%%%%%%%%%%%%%%%%%%%%%%

% Coriolis matrix C(q, dq)
C = zeros(7, 7);

% Define C matrix elements
C(1,3) = (m1 + m2) * (cos(theta1) * cos(theta2) * theta1_dot - sin(theta1) * sin(theta2) * theta2_dot);
C(1,4) = (m1 + m2) * (cos(theta1) * cos(theta2) * l1_dot - l1 * sin(theta1) * sin(theta2) * theta1_dot - l1 * cos(theta1) * sin(theta2) * theta2_dot);
C(1,5) = -(m1 + m2) * (sin(theta1) * sin(theta2) * l1_dot + l1 * cos(theta1) * sin(theta2) * theta1_dot + l1 * sin(theta1) * cos(theta2) * theta2_dot);
C(1,6) = -m2 * l2 * (sin(theta3) * cos(theta4) * theta3_dot + cos(theta3) * sin(theta4) * theta4_dot);
C(1,7) = -m2 * l2 * (cos(theta3) * sin(theta4) * theta3_dot + sin(theta3) * cos(theta4) * theta4_dot);

C(2,3) = (m1 + m2) * cos(theta2) * theta2_dot;
C(2,5) = (m1 + m2) * (cos(theta2) * l1_dot - l1 * sin(theta2) * theta2_dot);
C(2,7) = -m2 * l2 * sin(theta4) * theta4_dot;

C(3,4) = -(m1 + m2) * l1 * cos(theta2)^2 * theta1_dot;
C(3,5) = -(m1 + m2) * l1 * theta2_dot;
C(3,6) = -m2 * l2 * (cos(theta2) * cos(theta4) * cos(theta1 - theta3) * theta3_dot + cos(theta2) * sin(theta4) * sin(theta1 - theta3) * theta4_dot);
C(3,7) = -m2 * l2 * (cos(theta2) * sin(theta4) * theta3_dot + sin(theta2) * sin(theta4) * theta4_dot + cos(theta2) * cos(theta4) * cos(theta1 - theta3) * theta4_dot);

C(4,3) = (m1 + m2) * l1 * cos(theta2)^2 * theta1_dot;
C(4,4) = (m1 + m2) * (l1 * cos(theta2)^2 * l1_dot - l1^2 * sin(theta2) * cos(theta2) * theta2_dot);
C(4,5) = -(m1 + m2) * l1^2 * sin(theta2) * cos(theta2) * theta1_dot;
C(4,6) = m2 * l1 * l2 * (cos(theta2) * cos(theta4) * sin(theta1 - theta3) * theta3_dot + cos(theta2) * sin(theta4) * cos(theta1 - theta3) * theta4_dot);
C(4,7) = m2 * l1 * l2 * (cos(theta2) * cos(theta4) * sin(theta1 - theta3) * theta4_dot + cos(theta2) * sin(theta4) * cos(theta1 - theta3) * theta3_dot);

C(5,3) = (m1 + m2) * l1 * theta2_dot;
C(5,4) = (m1 + m2) * l1^2 * sin(theta2) * cos(theta2) * theta1_dot;
C(5,5) = (m1 + m2) * l1 * l1_dot;
C(5,6) = m2 * l1 * l2 * (sin(theta2) * cos(theta4) * cos(theta1 - theta3) * theta3_dot + sin(theta2) * sin(theta4) * sin(theta1 - theta3) * theta4_dot);
C(5,7) = m2 * l1 * l2 * (sin(theta2) * sin(theta4) * sin(theta1 - theta3) * theta3_dot + sin(theta2) * cos(theta4) * cos(theta1 - theta3) * theta4_dot ...
    - cos(theta2) * sin(theta4) * theta4_dot);

C(6,3) = m2 * l2 * (cos(theta2) * cos(theta4) * cos(theta1 - theta3) * theta1_dot - sin(theta2) * cos(theta4) * sin(theta1 - theta3) * theta2_dot);
C(6,4) = m2 * l2 * (cos(theta2) * cos(theta4) * cos(theta1 - theta3) * l1_dot - l1 * cos(theta2) * cos(theta4) * sin(theta1 - theta3) ...
    * theta1_dot - l1 * sin(theta2) * cos(theta4) * cos(theta1 - theta3) * theta2_dot);
C(6,5) = -m2 * l2 * (sin(theta2) * cos(theta4) * sin(theta1 - theta3) * l1_dot + l1 * sin(theta2) * cos(theta4) * cos(theta1 - theta3) ...
    * theta1_dot + l1 * cos(theta2) * cos(theta4) * sin(theta1 - theta3) * theta2_dot);
C(6,6) = -m2 * l2^2 * sin(theta4) * cos(theta4) * theta4_dot;
C(6,7) = -m2 * l2^2 * sin(theta4) * cos(theta4) * theta3_dot;

C(7,3) = m2 * l2 * (cos(theta2) * sin(theta4) * sin(theta1 - theta3) * theta1_dot + sin(theta2) * sin(theta4) * cos(theta1 - theta3) * theta2_dot ...
    + cos(theta2) * cos(theta4) * theta2_dot);
C(7,4) = m2 * l2 * (cos(theta2) * sin(theta4) * sin(theta1 - theta3) * l1_dot + l1 * cos(theta2) * sin(theta4) * cos(theta1 - theta3) ...
    * theta1_dot - l1 * sin(theta2) * sin(theta4) * sin(theta1 - theta3)*theta2_dot);
C(7,5) = m2 * l2 * (cos(theta2)*cos(theta4)*l1_dot + sin(theta2)*sin(theta4)*cos(theta1 - theta3)*l1_dot - l1 * sin(theta2)*sin(theta4)...
    *sin(theta1 - theta3)*theta1_dot + l1*cos(theta2)*sin(theta4)*cos(theta1 - theta3)*theta2_dot - l1*sin(theta2)*cos(theta4)*theta2_dot);
C(7,6) = m2 * l2^2 * sin(theta4) * cos(theta4) * theta3_dot;

% spliting

cxx = C(1:3, 1:3);
cxs = C(1:3, 4:7);
csx = C(4:7, 1:3);
css = C(4:7, 4:7);

%%%%%%%%%%%%%%%%%%%%%%%%%%%%%%%%%%%%%%%%%%%%%%%%%%%%%%%%%%%%%%%%%%%%%%%%%%%%%%%%%%%%%%%%%%%%%%%%%%%%%%%%%%%%%%%%%%%%%%%%%%%%%%%%%%%%%%%%%%%%%%%%%%%%%%%%%%%%%%%%%%%%%%%%%%%%%%%%%%%%%

% Gravity with friction matrix
G = zeros(7, 1);

% Define G matrix elements
G(1,1) = Frx;
G(2,1) = Fry;
G(3,1) = Frz - (m1 + m2) * g * cos(theta1) * cos(theta2);
% G(3,1) = 0;
G(4,1) = (m1 + m2) * g * l1 * sin(theta1) * cos(theta2);
G(5,1) = (m1 + m2) * g * l1 * cos(theta1) * sin(theta2);
G(6,1) = m2 * g * l2 * sin(theta3) * cos(theta4);
G(7,1) = m2 * g * l2 * cos(theta3) * sin(theta4);

% spliting

G1 = G(1:3);
G2 = G(4:7);

%%%%%%%%%%%%%%%%%%%%%%%%%%%%%%%%%%%%%%%%%%%%%%%%%%%%%%%%%%%%%%%%%%%%%%%%%%%%%%%%%%%%%%%%%%%%%%%%%%%%%%%%%%%%%%%%%%%%%%%%%%%%%%%%%%%%%%%%%%%%%%%%%%%%%%%%%%%%%%%%%%%%%%%%%%%%%%%%%%%%%%


end

== matlab function FBBSC_7dof/Subsystem5/MATLAB Function15 ==
  data: tau input; Fx output; Fy output
function [Fx, Fy] = fcn(tau)

Fx = tau(1);
Fy = tau(2);
end

== matlab function FBBSC_7dof/MATLAB Function17 ==
  data: U input size=[3 1]; tau output size=[3 1]; mxx input size=[3 3]; mxs input size=[3 4]; mss input size=[4 4]; msx input size=[4 3]; hx input size=[3 1]; hs input size=[4 1]
function tau  = fcn(U, mxx, mxs, mss, msx, hx, hs)

B = [1, 0, 0;
    0, 1, 0;
    0, 0, 1];

tau = inv(B'*B)*B'*((mxx - mxs*inv(mss)*msx)*U + (hx - mxs*inv(mss)*hs));


end

== matlab function FBBSC_7dof/MATLAB Function1 ==
  data: k1 input; K output; k2 input; k3 input
function K = fcn(k1, k2, k3)

K = [k1, 0, 0, 0;
    0, k2, 0, 0;
    0, 0, k3, 0];

end

== matlab function FBBSC_7dof/MATLAB Function16 ==
  settings: updateMethod=DISCRETE
  data: u input; y output
function y = fcn(u)
    persistent maxVal;
    
    % Check if maxVal is empty and initialize it if necessary
    if isempty(maxVal)
        maxVal = 0; % Initialize with negative infinity or another suitable value
    end
    
    % Update maxVal if the current input is greater
    if u > maxVal
        maxVal = u;
    end
    
    y = maxVal;
end

== matlab function FBBSC_7dof/MATLAB Function4 ==
  data: t input; m2 output
function m2 = fcn(t)

if t>=0 && t<3
    m2 = 0.6;
else
    m2 = 0.2;

% m2 = 0.6;


end

== matlab function FBBSC_7dof/MATLAB Function7 ==
  data: x_dot input; Frx output; y_dot input; Fry output; l1_dot input; Frz output
function [Frx, Fry, Frz] = fcn(x_dot, y_dot, l1_dot)

frox = 0.6;
froy = 0.6;
epsilon_x = 0.6;
epsilon_y = 0.6;
krx = 0.1;
kry = 0.1;
dz = 0.1;

Frx = frox*tanh(x_dot/epsilon_x) - krx*abs(x_dot)*x_dot;
Fry = froy*tanh(y_dot/epsilon_y) - kry*abs(y_dot)*y_dot;
Frz = dz * l1_dot;
end

== matlab function FBBSC_7dof/MATLAB Function2 ==
  settings: updateMethod=DISCRETE
  data: u input; y output
function y = fcn(u)
    persistent maxVal;
    
    % Check if maxVal is empty and initialize it if necessary
    if isempty(maxVal)
        maxVal = 0; % Initialize with negative infinity or another suitable value
    end
    
    % Update maxVal if the current input is greater
    if u > maxVal
        maxVal = u;
    end
    
    y = maxVal;
end

== matlab function FBBSC_7dof/MATLAB Function20 ==
  settings: updateMethod=DISCRETE
  data: u input; y output
function y = fcn(u)
    persistent maxVal;
    
    % Check if maxVal is empty and initialize it if necessary
    if isempty(maxVal)
        maxVal = 0; % Initialize with negative infinity or another suitable value
    end
    
    % Update maxVal if the current input is greater
    if u > maxVal
        maxVal = u;
    end
    
    y = maxVal;
end

== matlab function FBBSC_7dof/Subsystem5/MATLAB Function1 ==
  data: cxx input size=[2 2]; hx output size=[2 1]; cxs input size=[2 4]; G1 input size=[2 1]; csx input size=[4 2]; css input size=[4 4]; G2 input size=[4 1]; qx_dot input size=[2 1]; qs_dot input size=[4 1]; hs output size=[4 1]
function [hx, hs] = fcn(cxx, cxs, G1, csx, css, G2, qx_dot, qs_dot)

hx = cxx*qx_dot + cxs*qs_dot + G1;
hs = csx*qx_dot + css*qs_dot + G2;

end

== matlab function FBBSC_7dof/MATLAB Function ==
  data: Fx input; Fy input; Fz input; theta1 input; theta2 input; theta3 input; theta4 input; x_dot input; y_dot input; l1_dot input; theta1_dot input; theta2_dot input; theta3_dot input; theta4_dot input; m1 input; m2 input; M1 input; M2 input; l1 input; l2 input; q_ddot output size=[7 1]; Frx input; Fry input; Frz input
function q_ddot   = fcn(Fx, Fy, Fz, theta1, theta2, theta3, theta4,...
    x_dot, y_dot, l1_dot, theta1_dot, theta2_dot, theta3_dot, theta4_dot,...
    m1, m2, M1, M2, l1, l2, Frx, Fry, Frz)

g = 9.8;


% Mass matrix M(q)
M = zeros(7, 7);

% Define M matrix elements
M(1,1) = M1 + m1 + m2;
M(1,2) = 0;
M(1,3) = (m1 + m2) * sin(theta1) * cos(theta2);
M(1,4) = (m1 + m2) * l1 * cos(theta1) * cos(theta2);
M(1,5) = -(m1 + m2) * l1 * sin(theta1) * sin(theta2);
M(1,6) = m2 * l2 * cos(theta3) * cos(theta4);
M(1,7) = -m2 * l2 * sin(theta3) * sin(theta4);

M(2,1) = 0;
M(2,2) = M2 + m1 + m2;
M(2,3) = (m1 + m2) * sin(theta2);
M(2,4) = 0;
M(2,5) = (m1 + m2) * l1 * cos(theta2);
M(2,6) = 0;
M(2,7) = m2 * l2 * cos(theta4);

M(3,1) = (m1 + m2) * sin(theta1) * cos(theta2);
M(3,2) = (m1 + m2) * sin(theta2);
M(3,3) = m1 + m2;
M(3,4) = 0;
M(3,5) = 0;
M(3,6) = m2 * l2 * cos(theta2) * cos(theta4) * sin(theta1 - theta3);
M(3,7) = m2 * l2 * (sin(theta2) * cos(theta4) - cos(theta2) * sin(theta4) * cos(theta1 - theta3));

M(4,1) = (m1 + m2) * l1 * cos(theta1) * cos(theta2);
M(4,2) = 0;
M(4,3) = 0;
M(4,4) = (m1 + m2) * l1^2 * cos(theta2)^2;
M(4,5) = 0;
M(4,6) = m2*l1*l2*cos(theta2)*cos(theta4)*cos(theta1-theta3);
M(4,7) = m2*l1*l2*cos(theta2)*sin(theta4)*sin(theta1 - theta3);

M(5,1) = -(m1 + m2) * l1 * sin(theta1) * sin(theta2);
M(5,2) = (m1 + m2) * l1 * cos(theta2);
M(5,3) = 0;
M(5,4) = 0;
M(5,5) = (m1 + m2) * l1^2;
M(5,6) = -m2 * l1 * l2 * sin(theta2) * cos(theta4) * sin(theta1 - theta3);
M(5,7) = m2 * l1 * l2 * (cos(theta2) * cos(theta4) + sin(theta2) * sin(theta4) * cos(theta1 - theta3));

M(6,1) = m2 * l2 * cos(theta3) * cos(theta4);
M(6,2) = 0;
M(6,3) = m2 * l2 * cos(theta2) * cos(theta4) * sin(theta1 - theta3);
M(6,4) = m2*l1*l2*cos(theta2)*cos(theta4)*cos(theta1-theta3);
M(6,5) = -m2 * l1 * l2 * sin(theta2) * cos(theta4) * sin(theta1 - theta3);
M(6,6) = m2 * l2^2 * cos(theta4)^2;
M(6,7) = 0;

M(7,1) = -m2 * l2 * sin(theta3) * sin(theta4);
M(7,2) = m2 * l2 * cos(theta4);
M(7,3) = m2 * l2 * (sin(theta2) * cos(theta4) - cos(theta2) * sin(theta4) * cos(theta1 - theta3));
M(7,4) = m2*l1*l2*cos(theta2)*sin(theta4)*sin(theta1 - theta3);
M(7,5) = m2 * l1 * l2 * (cos(theta2) * cos(theta4) + sin(theta2) * sin(theta4) * cos(theta1 - theta3));
M(7,6) = 0;
M(7,7) = m2 * l2^2;

% Coriolis matrix C(q, dq)
C = zeros(7, 7);

% Define C matrix elements
C(1,3) = (m1 + m2) * (cos(theta1) * cos(theta2) * theta1_dot - sin(theta1) * sin(theta2) * theta2_dot);
C(1,4) = (m1 + m2) * (cos(theta1) * cos(theta2) * l1_dot - l1 * sin(theta1) * sin(theta2) * theta1_dot - l1 * cos(theta1) * sin(theta2) * theta2_dot);
C(1,5) = -(m1 + m2) * (sin(theta1) * sin(theta2) * l1_dot + l1 * cos(theta1) * sin(theta2) * theta1_dot + l1 * sin(theta1) * cos(theta2) * theta2_dot);
C(1,6) = -m2 * l2 * (sin(theta3) * cos(theta4) * theta3_dot + cos(theta3) * sin(theta4) * theta4_dot);
C(1,7) = -m2 * l2 * (cos(theta3) * sin(theta4) * theta3_dot + sin(theta3) * cos(theta4) * theta4_dot);

C(2,3) = (m1 + m2) * cos(theta2) * theta2_dot;
C(2,5) = (m1 + m2) * (cos(theta2) * l1_dot - l1 * sin(theta2) * theta2_dot);
C(2,7) = -m2 * l2 * sin(theta4) * theta4_dot;

C(3,4) = -(m1 + m2) * l1 * cos(theta2)^2 * theta1_dot;
C(3,5) = -(m1 + m2) * l1 * theta2_dot;
C(3,6) = -m2 * l2 * (cos(theta2) * cos(theta4) * cos(theta1 - theta3) * theta3_dot + cos(theta2) * sin(theta4) * sin(theta1 - theta3) * theta4_dot);
C(3,7) = -m2 * l2 * (cos(theta2) * sin(theta4) * theta3_dot + sin(theta2) * sin(theta4) * theta4_dot + cos(theta2) * cos(theta4) * cos(theta1 - theta3) * theta4_dot);

C(4,3) = (m1 + m2) * l1 * cos(theta2)^2 * theta1_dot;
C(4,4) = (m1 + m2) * (l1 * cos(theta2)^2 * l1_dot - l1^2 * sin(theta2) * cos(theta2) * theta2_dot);
C(4,5) = -(m1 + m2) * l1^2 * sin(theta2) * cos(theta2) * theta1_dot;
C(4,6) = m2 * l1 * l2 * (cos(theta2) * cos(theta4) * sin(theta1 - theta3) * theta3_dot + cos(theta2) * sin(theta4) * cos(theta1 - theta3) * theta4_dot);
C(4,7) = m2 * l1 * l2 * (cos(theta2) * cos(theta4) * sin(theta1 - theta3) * theta4_dot + cos(theta2) * sin(theta4) * cos(theta1 - theta3) * theta3_dot);

C(5,3) = (m1 + m2) * l1 * theta2_dot;
C(5,4) = (m1 + m2) * l1^2 * sin(theta2) * cos(theta2) * theta1_dot;
C(5,5) = (m1 + m2) * l1 * l1_dot;
C(5,6) = m2 * l1 * l2 * (sin(theta2) * cos(theta4) * cos(theta1 - theta3) * theta3_dot + sin(theta2) * sin(theta4) * sin(theta1 - theta3) * theta4_dot);
C(5,7) = m2 * l1 * l2 * (sin(theta2) * sin(theta4) * sin(theta1 - theta3) * theta3_dot + sin(theta2) * cos(theta4) * cos(theta1 - theta3) * theta4_dot ...
    - cos(theta2) * sin(theta4) * theta4_dot);

C(6,3) = m2 * l2 * (cos(theta2) * cos(theta4) * cos(theta1 - theta3) * theta1_dot - sin(theta2) * cos(theta4) * sin(theta1 - theta3) * theta2_dot);
C(6,4) = m2 * l2 * (cos(theta2) * cos(theta4) * cos(theta1 - theta3) * l1_dot - l1 * cos(theta2) * cos(theta4) * sin(theta1 - theta3) ...
    * theta1_dot - l1 * sin(theta2) * cos(theta4) * cos(theta1 - theta3) * theta2_dot);
C(6,5) = -m2 * l2 * (sin(theta2) * cos(theta4) * sin(theta1 - theta3) * l1_dot + l1 * sin(theta2) * cos(theta4) * cos(theta1 - theta3) ...
    * theta1_dot + l1 * cos(theta2) * cos(theta4) * sin(theta1 - theta3) * theta2_dot);
C(6,6) = -m2 * l2^2 * sin(theta4) * cos(theta4) * theta4_dot;
C(6,7) = -m2 * l2^2 * sin(theta4) * cos(theta4) * theta3_dot;

C(7,3) = m2 * l2 * (cos(theta2) * sin(theta4) * sin(theta1 - theta3) * theta1_dot + sin(theta2) * sin(theta4) * cos(theta1 - theta3) * theta2_dot ...
    + cos(theta2) * cos(theta4) * theta2_dot);
C(7,4) = m2 * l2 * (cos(theta2) * sin(theta4) * sin(theta1 - theta3) * l1_dot + l1 * cos(theta2) * sin(theta4) * cos(theta1 - theta3) ...
    * theta1_dot - l1 * sin(theta2) * sin(theta4) * sin(theta1 - theta3)*theta2_dot);
C(7,5) = m2 * l2 * (cos(theta2)*cos(theta4)*l1_dot + sin(theta2)*sin(theta4)*cos(theta1 - theta3)*l1_dot - l1 * sin(theta2)*sin(theta4)...
    *sin(theta1 - theta3)*theta1_dot + l1*cos(theta2)*sin(theta4)*cos(theta1 - theta3)*theta2_dot - l1*sin(theta2)*cos(theta4)*theta2_dot);
C(7,6) = m2 * l2^2 * sin(theta4) * cos(theta4) * theta3_dot;

% Gravity with friction matrix
G = zeros(7, 1);

% Define G matrix elements
G(1,1) = Frx;
G(2,1) = Fry;
G(3,1) = Frz - (m1 + m2) * g * cos(theta1) * cos(theta2);
% G(3,1) = 0;
G(4,1) = (m1 + m2) * g * l1 * sin(theta1) * cos(theta2);
G(5,1) = (m1 + m2) * g * l1 * cos(theta1) * sin(theta2);
G(6,1) = m2 * g * l2 * sin(theta3) * cos(theta4);
G(7,1) = m2 * g * l2 * cos(theta3) * sin(theta4);


q_dot = [x_dot; y_dot; l1_dot; theta1_dot; theta2_dot; theta3_dot; theta4_dot];
tau = [Fx; Fy; Fz; 0; 0; 0; 0];
D = tau - C*q_dot - G;

q_ddot = M\D;

end
